simulink model "linear_sys_est"  (R2021b)
settings: Solver=ode4  StartTime=0  StopTime=T_end  FixedStep=dt  RelTol=1e-3
values from neighbouring files (symbols this model uses):
  bias_Vx = 0.054595    [data.m]
  dt = 1e-3    (= 0.001)    [data.m]
  G_sens_y = 1    [data.m]
  IC = [0.0 0.0]    [data.m]    (also in postproc2.m)
  Kbbx = (mb * g * rb^2 * rm) / ((mb * rb^2 + Jb) * Ly)    (= 0.952057453416)    [data.m]
  Kbby = (mb * g * rb^2 * rm) / ((mb * rb^2 + Jb) * Lx)    (= 1.22502497502)    [data.m]
  PID_sim = PID(PID_idx(ii))    [postproc2.m]
  rate_limit = 20    [data.m]
  tau_mot_x = 0.066472    [data.m]
  tau_mot_y = 0.043174    [data.m]
  tau_sens_x = 0.025331    [data.m]
  tau_sens_y = 0.036103    [data.m]
  V2theta_x = 0.16565    [data.m]
  V2theta_y = 0.19677    [data.m]
undefined symbols (not defined in the file or in its folder): ref
libraries: slpidlib x2, simulink x1
settings Model: Creator=Daniele Oranges  LastModifiedBy=ernesto
settings DataIOCC: SaveFormat=StructureWithTime
settings OptimizationCC: BlockReduction=off  BufferReuse=off
settings DebuggingCC: AlgebraicLoopMsg=none  UnconnectedInputMsg=none  UnconnectedOutputMsg=none  UnconnectedLineMsg=none
settings ExplorerConfigSet: SimMechanicsOpenEditorOnUpdate=off

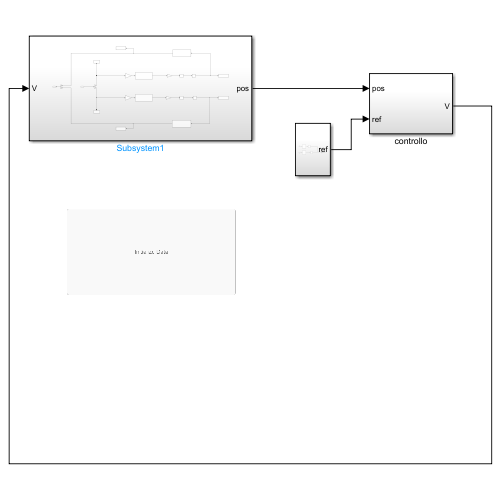
[thumbnail: Simulink's stored preview of the top-level diagram]
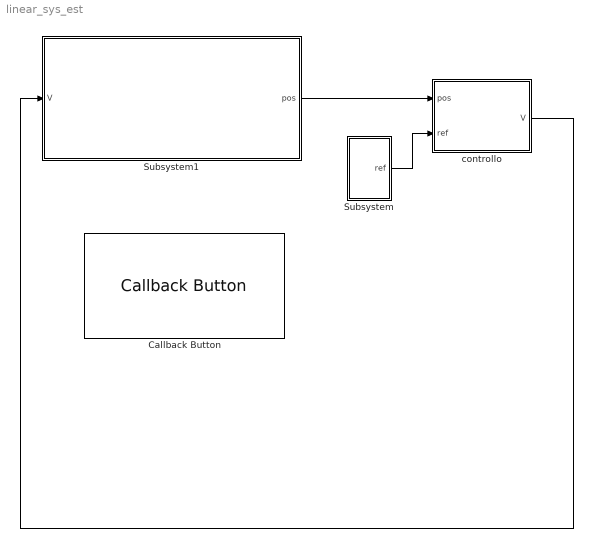
== system linear_sys_est ==
  Callback Button : CallbackButton  ButtonText=Initialize Data
      settings: ClickFcn=|
      | clear
      | data
  Subsystem : Subsystem
  Subsystem1 : Subsystem
  "controllo " : Subsystem
  wires:
  Subsystem/1(ref) -> "controllo "/2(ref)
  Subsystem1/1(pos) -> "controllo "/1("pos ")
  "controllo "/1(V) -> Subsystem1/1(V)

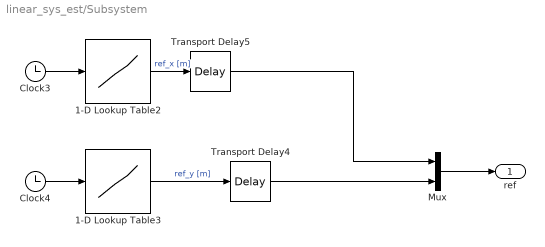
== system linear_sys_est/Subsystem ==
  1-D Lookup Table2 : Lookup_n-D  NumberOfTableDimensions=1  BreakpointsForDimension1=ref.x.t  Table=ref.x.v  InternalRulePriority=Speed  RndMeth=Simplest  InputSameDT=on
  1-D Lookup Table3 : Lookup_n-D  NumberOfTableDimensions=1  BreakpointsForDimension1=ref.y.t  Table=ref.y.v  InternalRulePriority=Speed  RndMeth=Simplest  InputSameDT=on
  Clock3 : Clock
  Clock4 : Clock
  Mux : Mux  Inputs=2
  Transport Delay4 : TransportDelay  DelayTime=dt
  Transport Delay5 : TransportDelay  DelayTime=dt
  ref : Outport
  wires:
  Transport Delay5/1 -> Mux/1
  1-D Lookup Table2/1 -> Transport Delay5/1  "ref_x [m]"
  1-D Lookup Table3/1 -> Transport Delay4/1  "ref_y [m]"
  Clock4/1 -> 1-D Lookup Table3/1
  Clock3/1 -> 1-D Lookup Table2/1
  Transport Delay4/1 -> Mux/2
  Mux/1 -> ref/1

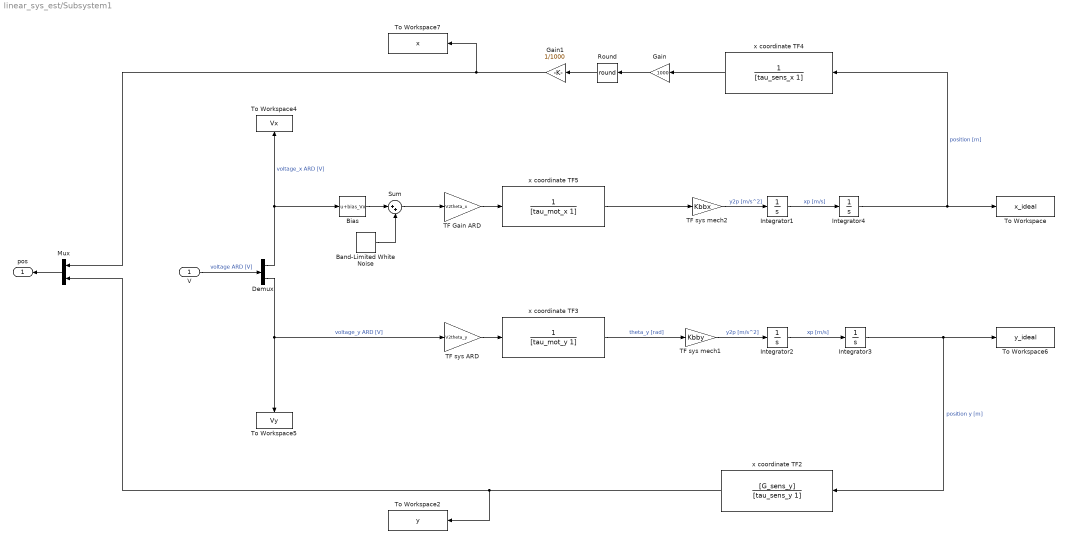
== system linear_sys_est/Subsystem1 ==
  V : Inport
  Band-Limited White Noise : simulink/Sources/Band-Limited White Noise  Cov=Ntension  Ts=dt  seed=[23341]
  Bias : Bias  Bias=bias_Vx
  Demux : Demux  Outputs=2
  Gain : Gain  Gain=1000
  Gain1 : Gain  Gain=1/1000
  Integrator1 : Integrator
  Integrator2 : Integrator
  Integrator3 : Integrator  InitialCondition=IC(2)
  Integrator4 : Integrator  InitialCondition=IC(1)
  Mux : Mux  Inputs=2
  Round : Rounding  Operator=round
  Sum : Sum  Inputs=|++
  TF Gain ARD : Gain  Gain=V2theta_x
  TF sys ARD : Gain  Gain=V2theta_y
  TF sys mech1 : Gain  Gain=Kbby
  TF sys mech2 : Gain  Gain=Kbbx
  To Workspace : ToWorkspace  VariableName=x_ideal  SaveFormat=Timeseries  SampleTime=-1
  To Workspace2 : ToWorkspace  VariableName=y  SaveFormat=Timeseries  SampleTime=-1
  To Workspace4 : ToWorkspace  VariableName=Vx  SaveFormat=Timeseries  SampleTime=-1
  To Workspace5 : ToWorkspace  VariableName=Vy  SaveFormat=Timeseries  SampleTime=-1
  To Workspace6 : ToWorkspace  VariableName=y_ideal  SaveFormat=Timeseries  SampleTime=-1
  To Workspace7 : ToWorkspace  VariableName=x  SaveFormat=Timeseries  SampleTime=-1
  x coordinate TF2 : TransferFcn  Numerator=[G_sens_y]  Denominator=[tau_sens_y 1]
  x coordinate TF3 : TransferFcn  Denominator=[tau_mot_y 1]
  x coordinate TF4 : TransferFcn  Denominator=[tau_sens_x 1]
  x coordinate TF5 : TransferFcn  Denominator=[tau_mot_x 1]
  pos : Outport
  wires:
  Demux/1 -> To Workspace4/1, Bias/1  "voltage_x ARD [V]"
  Integrator4/1 -> To Workspace/1, x coordinate TF4/1  "position [m]"
  Demux/2 -> To Workspace5/1, TF sys ARD/1  "voltage_y ARD [V]"
  Integrator3/1 -> To Workspace6/1, x coordinate TF2/1  "position y [m]"
  V/1 -> Demux/1  "voltage ARD [V]"
  Mux/1 -> pos/1
  x coordinate TF5/1 -> TF sys mech2/1
  TF Gain ARD/1 -> x coordinate TF5/1
  x coordinate TF3/1 -> TF sys mech1/1  "theta_y [rad]"
  TF sys ARD/1 -> x coordinate TF3/1
  Integrator2/1 -> Integrator3/1  "xp [m/s]"
  TF sys mech1/1 -> Integrator2/1  "y2p [m/s^2]"
  Integrator1/1 -> Integrator4/1  "xp [m/s]"
  TF sys mech2/1 -> Integrator1/1  "y2p [m/s^2]"
  x coordinate TF2/1 -> To Workspace2/1, Mux/2
  Gain/1 -> Round/1
  Round/1 -> Gain1/1
  x coordinate TF4/1 -> Gain/1
  Gain1/1 -> To Workspace7/1, Mux/1
  Bias/1 -> Sum/1
  Sum/1 -> TF Gain ARD/1
  Band-Limited White Noise/1 -> Sum/2

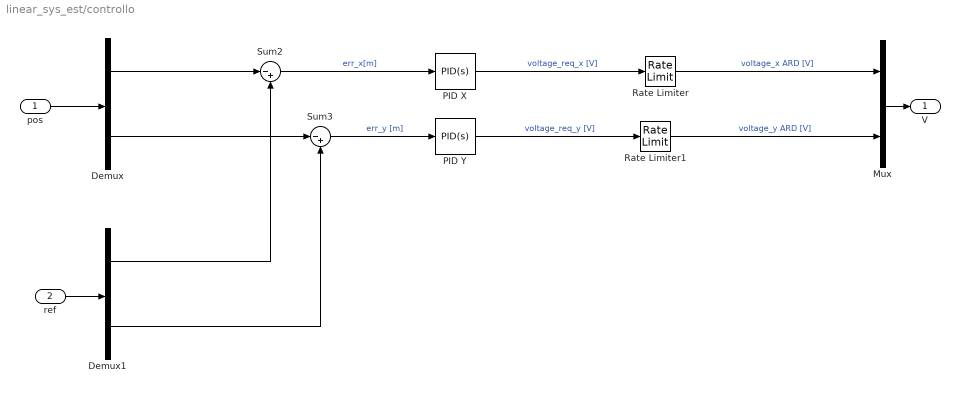
== system linear_sys_est/controllo  ==
  "pos " : Inport
  ref : Inport  Port=2
  Demux : Demux  Outputs=2
  Demux1 : Demux  Outputs=2
  Mux : Mux  Inputs=2
  PID X : slpidlib/PID Controller  Controller=PID  Form=Parallel  TimeDomain=Continuous-time  UseExternalTs=off  SampleTime=-1  IntegratorMethod=Forward Euler  FilterMethod=Forward Euler  ControllerParametersSource=internal  P=PID_sim.x.Kp  I=PID_sim.x.Ki  D=PID_sim.x.Kd  UseFilter=on  N=PID_sim.x.filter  TunerSelectOption=Transfer Function Based (PID Tuner App)  InitialConditionSource=internal  InitialConditionForIntegrator=0  InitialConditionForFilter=0  DifferentiatorICPrevScaledInput=0  ExternalReset=none  TrackingMode=off  Kt=1  LimitOutput=off  SatLimitsSource=internal  UpperSaturationLimit=inf  LowerSaturationLimit=-inf  LinearizeAsGain=on  AntiWindupMode=none  Kb=1  POutMin=[]  POutMax=[]  IOutMin=[]  IOutMax=[]  DOutMin=[]  DOutMax=[]  NOutMin=[]  NOutMax=[]  SumOutMin=[]  SumOutMax=[]  SaturationOutMin=[]  SaturationOutMax=[]  PParamMin=[]  PParamMax=[]  IParamMin=[]  IParamMax=[]  DParamMin=[]  DParamMax=[]  NParamMin=[]  NParamMax=[]  KbParamMin=[]  KbParamMax=[]  KtParamMin=[]  KtParamMax=[]  KbOutMin=[]  KbOutMax=[]  KtOutMin=[]  KtOutMax=[]  IntegratorOutMin=[]  IntegratorOutMax=[]  FilterOutMin=[]  FilterOutMax=[]  SumI1OutMin=[]  SumI1OutMax=[]  SumI2OutMin=[]  SumI2OutMax=[]  SumI3OutMin=[]  SumI3OutMax=[]  SumI4OutMin=[]  SumI4OutMax=[]  SumDOutMin=[]  SumDOutMax=[]  DifferentiatorOutMin=[]  DifferentiatorOutMax=[]  FilterDiffOutCoefMin=[]  FilterDiffOutCoefMax=[]  ReciprocalOutMin=[]  ReciprocalOutMax=[]  SumDenOutMin=[]  SumDenOutMax=[]  SumNumOutMin=[]  SumNumOutMax=[]  DivideOutMin=[]  DivideOutMax=[]  UdiffTsProdOutMin=[]  UdiffTsProdOutMax=[]  NTsProdOutMin=[]  NTsProdOutMax=[]  UintegralTsProdOutMin=[]  UintegralTsProdOutMax=[]  UngainTsProdOutMin=[]  UngainTsProdOutMax=[]  IntegratorContinuousStateAttributes=''  IntegratorStateMustResolveToSignalObject=off  IntegratorRTWStateStorageClass=Auto  FilterContinuousStateAttributes=''  FilterStateMustResolveToSignalObject=off  FilterRTWStateStorageClass=Auto  ParallelPVariant=InternalParameters  IdealPVariant=Disabled  IVariant=InternalParameters  DVariant=InternalParameters  IntegratorVariant=Continuous  SatVariant=Disabled  AWVariant=Passthrough  PCopyVariant=Disabled  TRVariant=Disabled  FdbkBlocksVariant=Forward  IdealPFdbkVariant=Disabled  SatFdbkVariant=Disabled  DerivativeFilterVariant=ContFilter  NVariant=InternalParameters  NCopyVariant=Disabled  FilterICVariant=InternalICsFilter  IntegratorICVariant=InternalICs  ExternalResetVariant=Disabled  TRSumVariant=Passthrough  SumFdbkVariant=Disabled  SumVariant=Sum_PID  TsampFilterVariant=InternalTs  TsampNgainVariant=Passthrough  TsampIntegralVariant=Passthrough  ExternalSaturationOutDataTypeStr=Inherit: Same as second input
  PID Y : slpidlib/PID Controller  Controller=PID  Form=Parallel  TimeDomain=Continuous-time  UseExternalTs=off  SampleTime=-1  IntegratorMethod=Forward Euler  FilterMethod=Forward Euler  ControllerParametersSource=internal  P=PID_sim.y.Kp  I=PID_sim.y.Ki  D=PID_sim.y.Kd  UseFilter=on  N=PID_sim.y.filter  TunerSelectOption=Transfer Function Based (PID Tuner App)  InitialConditionSource=internal  InitialConditionForIntegrator=0  InitialConditionForFilter=0  DifferentiatorICPrevScaledInput=0  ExternalReset=none  TrackingMode=off  Kt=1  LimitOutput=off  SatLimitsSource=internal  UpperSaturationLimit=inf  LowerSaturationLimit=-inf  LinearizeAsGain=on  AntiWindupMode=none  Kb=1  POutMin=[]  POutMax=[]  IOutMin=[]  IOutMax=[]  DOutMin=[]  DOutMax=[]  NOutMin=[]  NOutMax=[]  SumOutMin=[]  SumOutMax=[]  SaturationOutMin=[]  SaturationOutMax=[]  PParamMin=[]  PParamMax=[]  IParamMin=[]  IParamMax=[]  DParamMin=[]  DParamMax=[]  NParamMin=[]  NParamMax=[]  KbParamMin=[]  KbParamMax=[]  KtParamMin=[]  KtParamMax=[]  KbOutMin=[]  KbOutMax=[]  KtOutMin=[]  KtOutMax=[]  IntegratorOutMin=[]  IntegratorOutMax=[]  FilterOutMin=[]  FilterOutMax=[]  SumI1OutMin=[]  SumI1OutMax=[]  SumI2OutMin=[]  SumI2OutMax=[]  SumI3OutMin=[]  SumI3OutMax=[]  SumI4OutMin=[]  SumI4OutMax=[]  SumDOutMin=[]  SumDOutMax=[]  DifferentiatorOutMin=[]  DifferentiatorOutMax=[]  FilterDiffOutCoefMin=[]  FilterDiffOutCoefMax=[]  ReciprocalOutMin=[]  ReciprocalOutMax=[]  SumDenOutMin=[]  SumDenOutMax=[]  SumNumOutMin=[]  SumNumOutMax=[]  DivideOutMin=[]  DivideOutMax=[]  UdiffTsProdOutMin=[]  UdiffTsProdOutMax=[]  NTsProdOutMin=[]  NTsProdOutMax=[]  UintegralTsProdOutMin=[]  UintegralTsProdOutMax=[]  UngainTsProdOutMin=[]  UngainTsProdOutMax=[]  IntegratorContinuousStateAttributes=''  IntegratorStateMustResolveToSignalObject=off  IntegratorRTWStateStorageClass=Auto  FilterContinuousStateAttributes=''  FilterStateMustResolveToSignalObject=off  FilterRTWStateStorageClass=Auto  ParallelPVariant=InternalParameters  IdealPVariant=Disabled  IVariant=InternalParameters  DVariant=InternalParameters  IntegratorVariant=Continuous  SatVariant=Disabled  AWVariant=Passthrough  PCopyVariant=Disabled  TRVariant=Disabled  FdbkBlocksVariant=Forward  IdealPFdbkVariant=Disabled  SatFdbkVariant=Disabled  DerivativeFilterVariant=ContFilter  NVariant=InternalParameters  NCopyVariant=Disabled  FilterICVariant=InternalICsFilter  IntegratorICVariant=InternalICs  ExternalResetVariant=Disabled  TRSumVariant=Passthrough  SumFdbkVariant=Disabled  SumVariant=Sum_PID  TsampFilterVariant=InternalTs  TsampNgainVariant=Passthrough  TsampIntegralVariant=Passthrough  ExternalSaturationOutDataTypeStr=Inherit: Same as second input
  Rate Limiter : RateLimiter  RisingSlewLimit=rate_limit  FallingSlewLimit=-rate_limit  SampleTimeMode=inherited
  Rate Limiter1 : RateLimiter  RisingSlewLimit=rate_limit  FallingSlewLimit=-rate_limit  SampleTimeMode=inherited
  Sum2 : Sum  Inputs=|-+
  Sum3 : Sum  Inputs=|-+
  V : Outport
  wires:
  "pos "/1 -> Demux/1
  Mux/1 -> V/1
  Demux/1 -> Sum2/1
  Demux/2 -> Sum3/1
  PID X/1 -> Rate Limiter/1  "voltage_req_x [V]"
  Rate Limiter/1 -> Mux/1  "voltage_x ARD [V]"
  Sum2/1 -> PID X/1  "err_x[m]"
  Rate Limiter1/1 -> Mux/2  "voltage_y ARD [V]"
  Sum3/1 -> PID Y/1  "err_y [m]"
  PID Y/1 -> Rate Limiter1/1  "voltage_req_y [V]"
  Demux1/1 -> Sum2/2
  Demux1/2 -> Sum3/2
  ref/1 -> Demux1/1
